simulink model "ModeloQuadrotor"  (R2023b)
settings: Solver=VariableStepAuto  StartTime=0.0  StopTime=10.0  RelTol=1e-3
undefined symbols (not defined in the file): a, A_drag, b, B_drag, g, Ixx, Iyy, Izz, K, L, m, Po
settings Model: Creator=juanr  LastModifiedBy=juanr

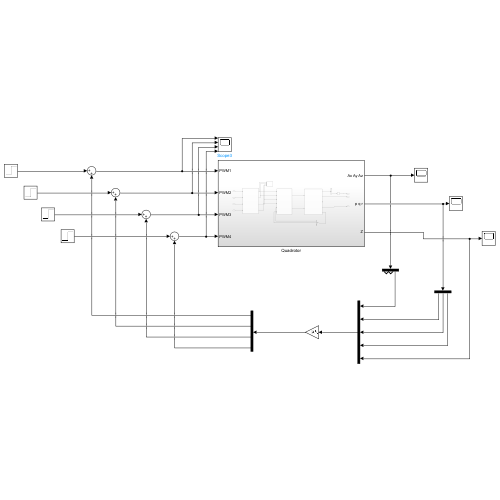
[thumbnail: Simulink's stored preview of the top-level diagram]
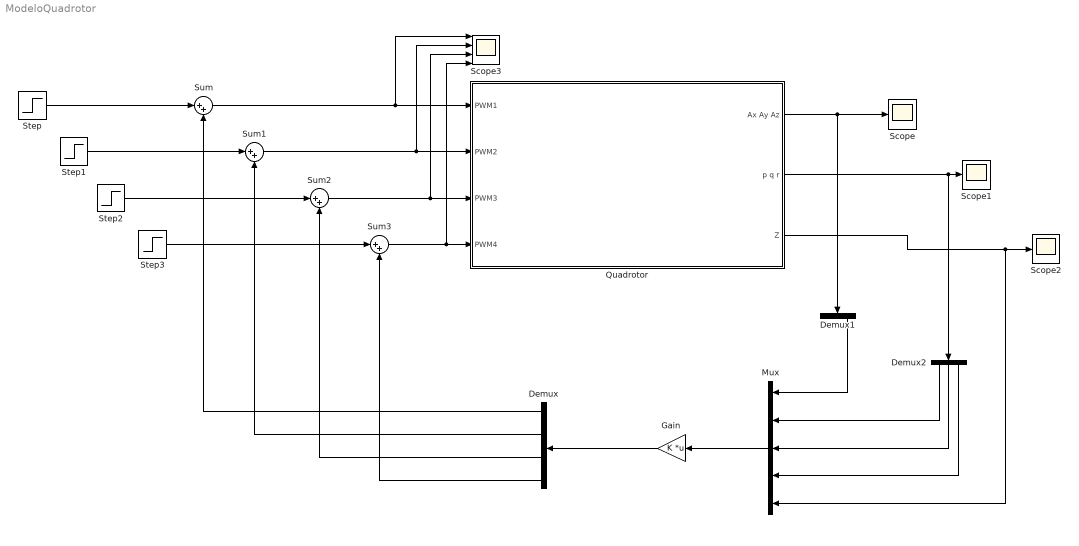
== system ModeloQuadrotor ==
  Demux : Demux
  Demux1 : Demux  Outputs=3
  Demux2 : Demux  Outputs=3
  Gain : Gain  Gain=K  Multiplication=Matrix(K*u)
  Mux : Mux  Inputs=5
  Quadrotor : Subsystem
  Scope : Scope
  Scope1 : Scope
  Scope2 : Scope
  Scope3 : Scope  NumInputPorts=4
  Step{,1..3} (4 alike) : Step  Time=0  After=Po  SampleTime=0
  Sum{,1..3} (4 alike) : Sum  Inputs=|++
  wires:
  Quadrotor/1(Ax Ay Az) -> Demux1/1, Scope/1
  Quadrotor/2(p q r) -> Demux2/1, Scope1/1
  Quadrotor/3(Z) -> Mux/5, Scope2/1
  Step/1 -> Sum/1
  Sum/1 -> Scope3/1, Quadrotor/1(PWM1)
  Sum1/1 -> Scope3/2, Quadrotor/2(PWM2)
  Sum2/1 -> Scope3/3, Quadrotor/3(PWM3)
  Sum3/1 -> Scope3/4, Quadrotor/4(PWM4)
  Step1/1 -> Sum1/1
  Step2/1 -> Sum2/1
  Step3/1 -> Sum3/1
  Gain/1 -> Demux/1
  Mux/1 -> Gain/1
  Demux1/3 -> Mux/1
  Demux2/1 -> Mux/2
  Demux2/2 -> Mux/3
  Demux2/3 -> Mux/4
  Demux/1 -> Sum/2
  Demux/2 -> Sum1/2
  Demux/3 -> Sum2/2
  Demux/4 -> Sum3/2

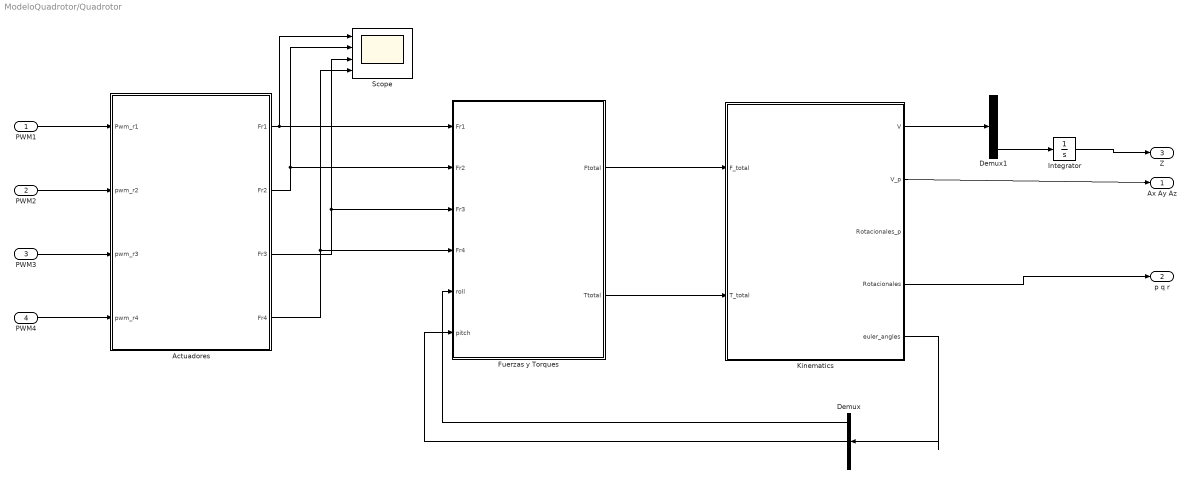
== system ModeloQuadrotor/Quadrotor ==
  PWM1 : Inport
  PWM2 : Inport  Port=2
  PWM3 : Inport  Port=3
  PWM4 : Inport  Port=4
  Actuadores : Subsystem
  Demux : Demux  Outputs=3
  Demux1 : Demux  Outputs=3
  Fuerzas y Torques : Subsystem
  Integrator : Integrator
  Kinematics : Subsystem
  Scope : Scope  NumInputPorts=4
  Ax Ay Az : Outport
  p q r : Outport  Port=2
  Z : Outport  Port=3
  wires:
  PWM1/1 -> Actuadores/1(Pwm_r1)
  PWM2/1 -> Actuadores/2(pwm_r2)
  PWM3/1 -> Actuadores/3(pwm_r3)
  PWM4/1 -> Actuadores/4(pwm_r4)
  Actuadores/1(Fr1) -> Fuerzas y Torques/1(Fr1), Scope/1
  Actuadores/2(Fr2) -> Fuerzas y Torques/2(Fr2), Scope/2
  Actuadores/3(Fr3) -> Fuerzas y Torques/3(Fr3), Scope/3
  Actuadores/4(Fr4) -> Fuerzas y Torques/4(Fr4), Scope/4
  Fuerzas y Torques/1(Ftotal) -> Kinematics/1(F_total)
  Fuerzas y Torques/2(Ttotal) -> Kinematics/2(T_total)
  Demux/1 -> Fuerzas y Torques/5(roll)
  Demux/2 -> Fuerzas y Torques/6(pitch)
  Kinematics/5(euler_angles) -> Demux/1
  Kinematics/4(Rotacionales) -> p q r/1
  Kinematics/1(V) -> Demux1/1
  Demux1/3 -> Integrator/1
  Integrator/1 -> Z/1
  Kinematics/2(V_p) -> Ax Ay Az/1

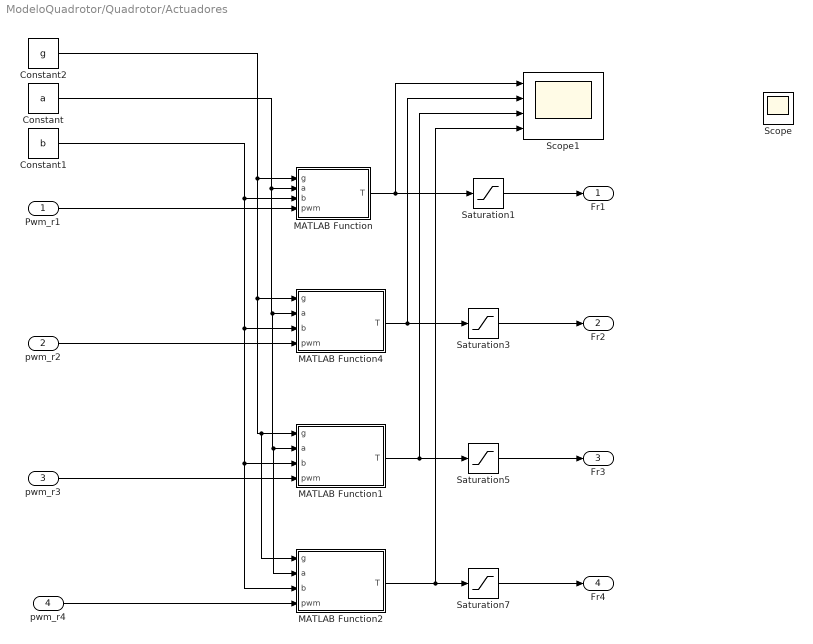
== system ModeloQuadrotor/Quadrotor/Actuadores ==
  Pwm_r1 : Inport
  pwm_r2 : Inport  Port=2
  pwm_r3 : Inport  Port=3
  pwm_r4 : Inport  Port=4
  Constant : Constant  Value=a
  Constant1 : Constant  Value=b
  Constant2 : Constant  Value=g
  MATLAB Function : MATLAB Function  TreatAsAtomicUnit=on
  MATLAB Function1 : MATLAB Function  TreatAsAtomicUnit=on
  MATLAB Function2 : MATLAB Function  TreatAsAtomicUnit=on
  MATLAB Function4 : MATLAB Function  TreatAsAtomicUnit=on
  Saturation{1,3,5,7} (4 alike) : Saturate  UpperLimit=10  LowerLimit=0  ZeroCross=off
  Scope : Scope
  Scope1 : Scope  NumInputPorts=4
  Fr1 : Outport
  Fr2 : Outport  Port=2
  Fr3 : Outport  Port=3
  Fr4 : Outport  Port=4
  wires:
  Pwm_r1/1 -> MATLAB Function/4(pwm)
  Constant/1 -> MATLAB Function4/2(a), MATLAB Function2/2(a), MATLAB Function1/2(a), MATLAB Function/2(a)
  Constant1/1 -> MATLAB Function4/3(b), MATLAB Function2/3(b), MATLAB Function1/3(b), MATLAB Function/3(b)
  MATLAB Function/1(T) -> Scope1/1, Saturation1/1
  MATLAB Function4/1(T) -> Scope1/2, Saturation3/1
  pwm_r2/1 -> MATLAB Function4/4(pwm)
  pwm_r3/1 -> MATLAB Function1/4(pwm)
  pwm_r4/1 -> MATLAB Function2/4(pwm)
  Saturation1/1 -> Fr1/1
  Saturation3/1 -> Fr2/1
  Saturation5/1 -> Fr3/1
  Saturation7/1 -> Fr4/1
  Constant2/1 -> MATLAB Function2/1(g), MATLAB Function1/1(g), MATLAB Function4/1(g), MATLAB Function/1(g)
  MATLAB Function1/1(T) -> Scope1/3, Saturation5/1
  MATLAB Function2/1(T) -> Scope1/4, Saturation7/1

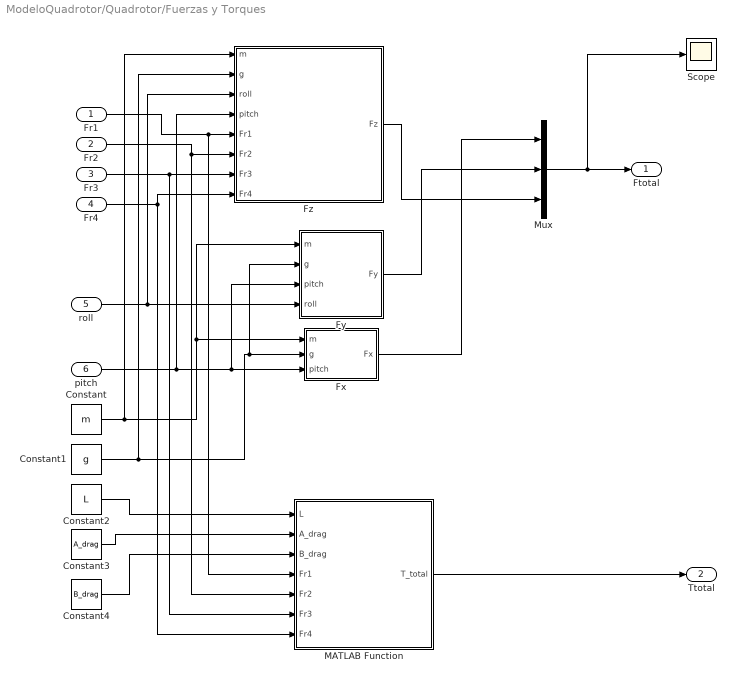
== system ModeloQuadrotor/Quadrotor/Fuerzas y Torques ==
  Fr1 : Inport
  Fr2 : Inport  Port=2
  Fr3 : Inport  Port=3
  Fr4 : Inport  Port=4
  roll : Inport  Port=5
  pitch : Inport  Port=6
  Constant : Constant  Value=m
  Constant1 : Constant  Value=g
  Constant2 : Constant  Value=L
  Constant3 : Constant  Value=A_drag
  Constant4 : Constant  Value=B_drag
  Fx : MATLAB Function  TreatAsAtomicUnit=on
  Fy : MATLAB Function  TreatAsAtomicUnit=on
  Fz : MATLAB Function  TreatAsAtomicUnit=on
  MATLAB Function : MATLAB Function  TreatAsAtomicUnit=on
  Mux : Mux  Inputs=3
  Scope : Scope
  Ftotal : Outport
  Ttotal : Outport  Port=2
  wires:
  pitch/1 -> Fz/4(pitch), Fy/3(pitch), Fx/3(pitch)
  Constant/1 -> Fz/1(m), Fy/1(m), Fx/1(m)
  Constant1/1 -> Fz/2(g), Fy/2(g), Fx/2(g)
  roll/1 -> Fz/3(roll), Fy/4(roll)
  Fr4/1 -> Fz/8(Fr4), MATLAB Function/7(Fr4)
  Fr3/1 -> MATLAB Function/6(Fr3), Fz/7(Fr3)
  Fr2/1 -> MATLAB Function/5(Fr2), Fz/6(Fr2)
  Fr1/1 -> MATLAB Function/4(Fr1), Fz/5(Fr1)
  Fx/1(Fx) -> Mux/1
  Fy/1(Fy) -> Mux/2
  Fz/1(Fz) -> Mux/3
  Mux/1 -> Scope/1, Ftotal/1
  MATLAB Function/1(T_total) -> Ttotal/1
  Constant2/1 -> MATLAB Function/1(L)
  Constant3/1 -> MATLAB Function/2(A_drag)
  Constant4/1 -> MATLAB Function/3(B_drag)

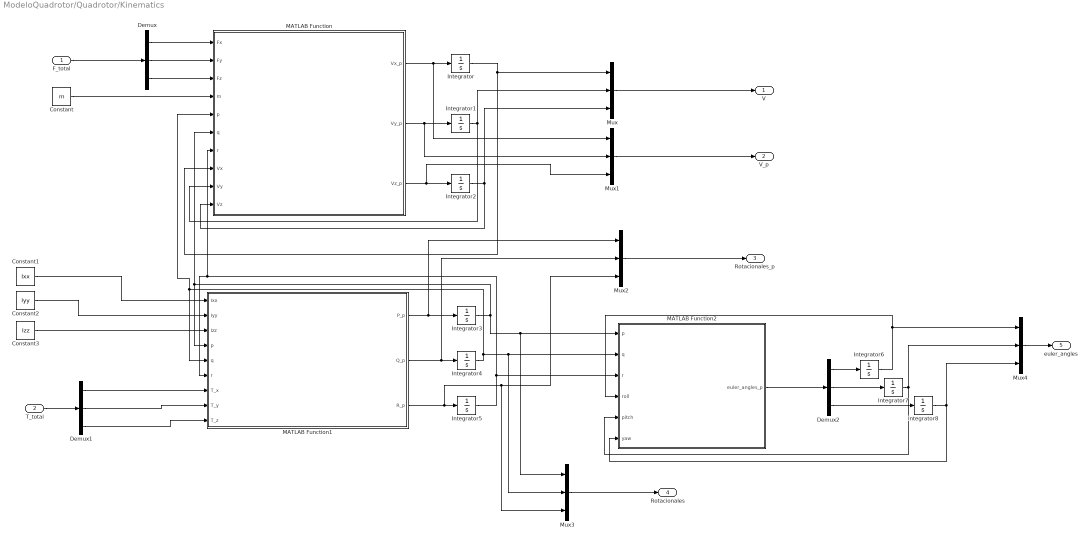
== system ModeloQuadrotor/Quadrotor/Kinematics ==
  F_total : Inport
  T_total : Inport  Port=2
  Constant : Constant  Value=m
  Constant1 : Constant  Value=Ixx
  Constant2 : Constant  Value=Iyy
  Constant3 : Constant  Value=Izz
  Demux : Demux  Outputs=3
  Demux1 : Demux  Outputs=3
  Demux2 : Demux  Outputs=3
  Integrator{,1..8} (9 alike) : Integrator
  MATLAB Function : MATLAB Function  TreatAsAtomicUnit=on
  MATLAB Function1 : MATLAB Function  TreatAsAtomicUnit=on
  MATLAB Function2 : MATLAB Function  TreatAsAtomicUnit=on
  Mux{,1..4} (5 alike) : Mux  Inputs=3
  V : Outport
  V_p : Outport  Port=2
  Rotacionales_p : Outport  Port=3
  Rotacionales : Outport  Port=4
  euler_angles : Outport  Port=5
  wires:
  F_total/1 -> Demux/1
  Demux/1 -> MATLAB Function/1(Fx)
  Demux/2 -> MATLAB Function/2(Fy)
  Demux/3 -> MATLAB Function/3(Fz)
  Constant/1 -> MATLAB Function/4(m)
  MATLAB Function/1(Vx_p) -> Mux1/1, Integrator/1
  MATLAB Function/2(Vy_p) -> Mux1/2, Integrator1/1
  MATLAB Function/3(Vz_p) -> Mux1/3, Integrator2/1
  Integrator2/1 -> Mux/3, MATLAB Function/10(Vz)
  Integrator1/1 -> MATLAB Function/9(Vy), Mux/2
  Integrator/1 -> MATLAB Function/8(Vx), Mux/1
  Demux1/1 -> MATLAB Function1/7(T_x)
  Demux1/2 -> MATLAB Function1/8(T_y)
  Demux1/3 -> MATLAB Function1/9(T_z)
  T_total/1 -> Demux1/1
  Constant1/1 -> MATLAB Function1/1(Ixx)
  Constant2/1 -> MATLAB Function1/2(Iyy)
  Constant3/1 -> MATLAB Function1/3(Izz)
  MATLAB Function1/1(P_p) -> Mux2/1, Integrator3/1
  MATLAB Function1/2(Q_p) -> Mux2/2, Integrator4/1
  MATLAB Function1/3(R_p) -> Mux3/3, Mux2/3, Integrator5/1
  Integrator3/1 -> Mux3/1, MATLAB Function2/1(p), MATLAB Function/6(q), MATLAB Function1/4(p)
  Integrator4/1 -> Mux3/2, MATLAB Function2/2(q), MATLAB Function1/5(q), MATLAB Function/5(p)
  Integrator5/1 -> MATLAB Function2/3(r), MATLAB Function/7(r), MATLAB Function1/6(r)
  MATLAB Function2/1(euler_angles_p) -> Demux2/1
  Demux2/1 -> Integrator6/1
  Demux2/2 -> Integrator7/1
  Demux2/3 -> Integrator8/1
  Integrator8/1 -> MATLAB Function2/6(yaw), Mux4/3
  Integrator7/1 -> MATLAB Function2/5(pitch), Mux4/2
  Integrator6/1 -> Mux4/1, MATLAB Function2/4(roll)
  Mux/1 -> V/1
  Mux1/1 -> V_p/1
  Mux2/1 -> Rotacionales_p/1
  Mux3/1 -> Rotacionales/1
  Mux4/1 -> euler_angles/1

== matlab function ModeloQuadrotor/Quadrotor/Kinematics/MATLAB Function ==
  data: Fx input; Vx_p output; Fy input; Fz input; m input; p input; q input; r input; Vx input; Vy input; Vz input; Vy_p output; Vz_p output
function [Vx_p, Vy_p, Vz_p] = fcn(Fx, Fy, Fz, m, p, q, r, Vx, Vy, Vz)

Vx_p = 1/m*(Fx-(q*Vz-r*Vy));
Vy_p = 1/m*(Fy-(r*Vx-Vz*p));
Vz_p = 1/m*(Fz-(p*Vz-q*Vx));

== matlab function ModeloQuadrotor/Quadrotor/Kinematics/MATLAB Function1 ==
  data: Ixx input; P_p output; Iyy input; Izz input; p input; q input; r input; T_x input; T_y input; T_z input; Q_p output; R_p output
function [P_p, Q_p, R_p] = fcn(Ixx, Iyy, Izz, p, q, r, T_x, T_y, T_z)

%% Los torques se nombran como
%T_x = L
%T_y = M
%T_z = N

P_p = 1/Ixx*(T_x-(Izz-Iyy)*q*r);
Q_p = 1/Iyy*(T_y-(Ixx-Izz)*p*r);
R_p = 1/Izz*(T_z-(Iyy-Ixx)*p*q);

== matlab function ModeloQuadrotor/Quadrotor/Kinematics/MATLAB Function2 ==
  data: p input; euler_angles_p output; q input; r input; roll input; pitch input; yaw input
function euler_angles_p = fcn(p, q, r, roll, pitch, yaw)

euler_angles_p = [1, sin(roll)* tan(pitch), cos(roll)*tan(pitch);
        0, cos(roll), -sin(roll);
        0, -sin(roll)/cos(pitch), cos(roll)/cos(pitch)]*[p;q;r];

== matlab function ModeloQuadrotor/Quadrotor/Actuadores/MATLAB Function1 ==
  data: g input; a input; b input; pwm input; T output
function T = fcn(g,a,b,pwm)

T = (a*pwm+b)*g;

== matlab function ModeloQuadrotor/Quadrotor/Actuadores/MATLAB Function ==
  data: g input; a input; b input; pwm input; T output
function T = fcn(g,a,b,pwm)

T = (a*pwm+b)*g;

== matlab function ModeloQuadrotor/Quadrotor/Actuadores/MATLAB Function2 ==
  data: g input; a input; b input; pwm input; T output
function T = fcn(g,a,b,pwm)

T = (a*pwm+b)*g;

== matlab function ModeloQuadrotor/Quadrotor/Fuerzas y Torques/Fx ==
  data: m input; Fx output; g input; pitch input
function Fx = fcn(m,g,pitch)

Fx = -m*g*sin(pitch);

== matlab function ModeloQuadrotor/Quadrotor/Actuadores/MATLAB Function4 ==
  data: g input; a input; b input; pwm input; T output
function T = fcn(g,a,b,pwm)

T = (a*pwm+b)*g;

== matlab function ModeloQuadrotor/Quadrotor/Fuerzas y Torques/Fy ==
  data: m input; Fy output; g input; pitch input; roll input
function Fy = fcn(m,g,pitch,roll)

Fy = m*g*sin(roll)*cos(pitch);

== matlab function ModeloQuadrotor/Quadrotor/Fuerzas y Torques/Fz ==
  data: m input; Fz output; g input; roll input; pitch input; Fr1 input; Fr2 input; Fr3 input; Fr4 input
function Fz = fcn(m,g,roll,pitch,Fr1, Fr2, Fr3, Fr4)

Fz = (Fr1+Fr2+Fr3+Fr4)-(m*g*cos(roll)*cos(pitch));

== matlab function ModeloQuadrotor/Quadrotor/Fuerzas y Torques/MATLAB Function ==
  data: L input; A_drag input; B_drag input; T_total output; Fr1 input; Fr2 input; Fr3 input; Fr4 input
function T_total  = fcn(L, A_drag, B_drag, Fr1, Fr2, Fr3, Fr4)

%
%Fri Corresponde a las Fuerzas de cada uno de los rotores
%

Tr1=[L*Fr1;0;0];
Tr2=[0;-L*Fr2;0];
Tr3=[-L*Fr3;0;0];
Tr4=[0;L*Fr4;0];

Qd1=A_drag*(Fr1^(1.5))+B_drag;
Qd2=A_drag*(Fr2^(1.5))+B_drag;
Qd3=A_drag*(Fr3^(1.5))+B_drag;
Qd4=A_drag*(Fr4^(1.5))+B_drag;

Td1=[0;0;Qd1];
Td2=[0;0;Qd2];
Td3=[0;0;Qd3];
Td4=[0;0;Qd4];

T_total = ((Tr1-Td1)+(Tr3-Td3))-((Tr2-Td2)+(Tr4-Td4));
